simulink model "LabB_CheckCommunications"  (R2025b)
settings: Solver=FixedStepDiscrete  StartTime=0.0  StopTime=Inf  FixedStep=fSamplingPeriod  RelTol=1e-3  EnableMultiTasking=on
values from neighbouring files (symbols this model uses):
  fSamplingPeriod = 0.01    [GetDataFromSerial.m]    (also in GetRuns.m = 0.005; LabA_Solutions_LoadPhysicalParameters.m = 1 / sampling_freq; LabA_solutions.m = 1 / sampling_freq; LabB_ObserverAndControllerOverRobot_Parameters.m = 0.005)
undefined symbols (not defined in the file or in its folder): DiscIntNeverNeededParam
libraries: simulink_extras x3, arduinolib x3, xpcutilitieslib x1, MinSegLibrary_M2V3 x1
settings Model: SimulationMode=external  ExtModeTrigDuration=2  Creator=Alec  LastModifiedBy=emil
settings SolverCC: AlgebraicLoopSolver=TrustRegion
settings DataIOCC: LimitDataPoints=on  SaveFormat=Array  ReturnWorkspaceOutputs=off
settings OptimizationCC: PassReuseOutputArgsAs=Individual arguments  ExpressionDepthLimit=2147483647.0  MaxStackSize=64  EfficientTunableParamExpr=on
settings DebuggingCC: UnderspecifiedInitializationDetection=Classic  MergeDetectMultiDrivingBlocksExec=none  ParameterTunabilityLossMsg=error  UnconnectedInputMsg=warning  UnconnectedOutputMsg=warning  UnconnectedLineMsg=warning  StateNameClashWarn=warning  SFUnexpectedBacktrackingDiag=warning  SFNoUnconditionalDefaultTransitionDiag=warning  SFExecutionAtInitializationDiag=none  ArithmeticOperatorsInVariantConditions=warning
settings HardwareCC: ProdBitPerInt=16.0  ProdBitPerPointer=16.0  ProdBitPerSizeT=16.0  ProdBitPerPtrDiffT=16.0  ProdLargestAtomicFloat=None  ProdWordSize=8.0  ProdHWDeviceType=Atmel->AVR
settings ModelReferenceCC: EnableRefExpFcnMdlSchedulingChecks=on  PropagateSignalLabelsOutOfModel=off
settings SFSimCC: SimUseLocalCustomCode=off  MATLABDynamicMemAlloc=off  CustomCodeUndefinedFunction=UseInterfaceOnly
settings RTWCC: SystemTargetFile=ert.tlc  HardwareBoard=Arduino Mega 2560  TemplateMakefile=ert_default_tmf  GenerateReport=on  RTWVerbose=off  RTWUseLocalCustomCode=off  Toolchain=Arduino AVR  BuildConfiguration=Faster Runs  IncludeHyperlinkInReport=on  LaunchReport=on  GenerateTraceInfo=on  GenerateTraceReport=on  GenerateTraceReportSl=on  GenerateTraceReportSf=on  GenerateTraceReportEml=on  GPUComputeCapability=3.5  Description=Embedded Coder
settings CodeAppCC: ForceParamTrailComments=on  IgnoreCustomStorageClasses=off  OperatorAnnotations=on  SimulinkDataObjDesc=on  SFDataObjDesc=on  MATLABFcnDesc=on  CustomSymbolStrType=$N$R$M  InsertBlockDesc=on  StateflowObjectComments=on  MATLABSourceComments=on  InternalIdentifier=Classic
settings ERTTargetCC: InlinedParameterPlacement=Hierarchical  DynamicArrayContainerType=coder::array  SupportContinuousTime=on  SupportVariableSizeSignals=on
settings ConfigComp: CovMetricSettings=dw  CovSaveCumulativeToWorkspaceVar=on  CovSaveSingleToWorkspaceVar=on  CovExternalEMLEnable=off

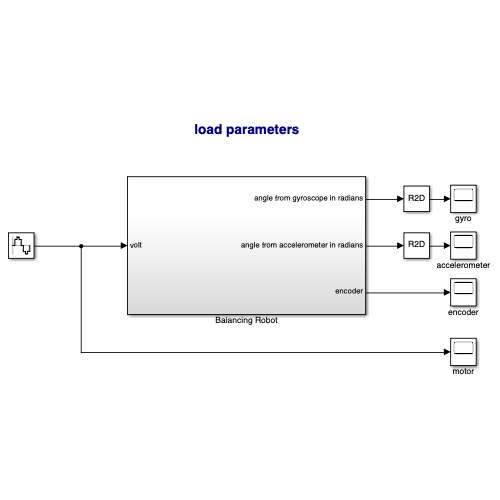
[thumbnail: Simulink's stored preview of the top-level diagram]
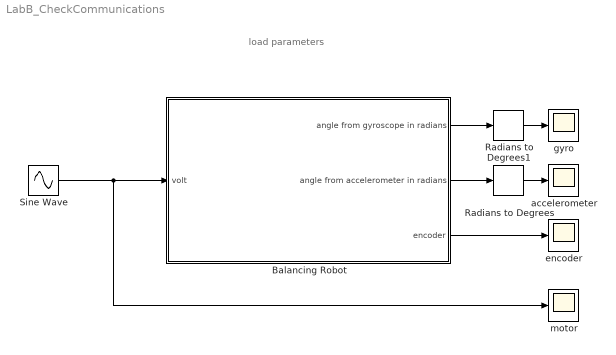
== system LabB_CheckCommunications ==
  note: load parameters
  Balancing Robot : Subsystem
  Radians to Degrees : simulink_extras/Transformations/Radians to Degrees
  Radians to Degrees1 : simulink_extras/Transformations/Radians to Degrees
  Sine Wave : Sin  Frequency=5  SampleTime=fSamplingPeriod
  accelerometer : Scope
      settings: ActiveDisplayYMinimum=-45  ActiveDisplayYMaximum=30  DataLoggingVariableName=tAngleFromAccelerometer
  encoder : Scope
      settings: TimeSpan=10  ActiveDisplayYMinimum=-268.25  ActiveDisplayYMaximum=-125.75  DataLoggingVariableName=tEncoder
  gyro : Scope
      settings: ActiveDisplayYMinimum=16.70976  ActiveDisplayYMaximum=26.00492  DataLoggingVariableName=tAngleFromGyro
  motor : Scope
      settings: ActiveDisplayYMinimum=-1  ActiveDisplayYMaximum=1  DataLoggingVariableName=tMotor
  wires:
  Balancing Robot/1(angle from gyroscope in radians) -> Radians to Degrees1/1
  Balancing Robot/2(angle from accelerometer in radians) -> Radians to Degrees/1
  Balancing Robot/3(encoder) -> encoder/1
  Radians to Degrees1/1 -> gyro/1
  Radians to Degrees/1 -> accelerometer/1
  Sine Wave/1 -> motor/1, Balancing Robot/1(volt)

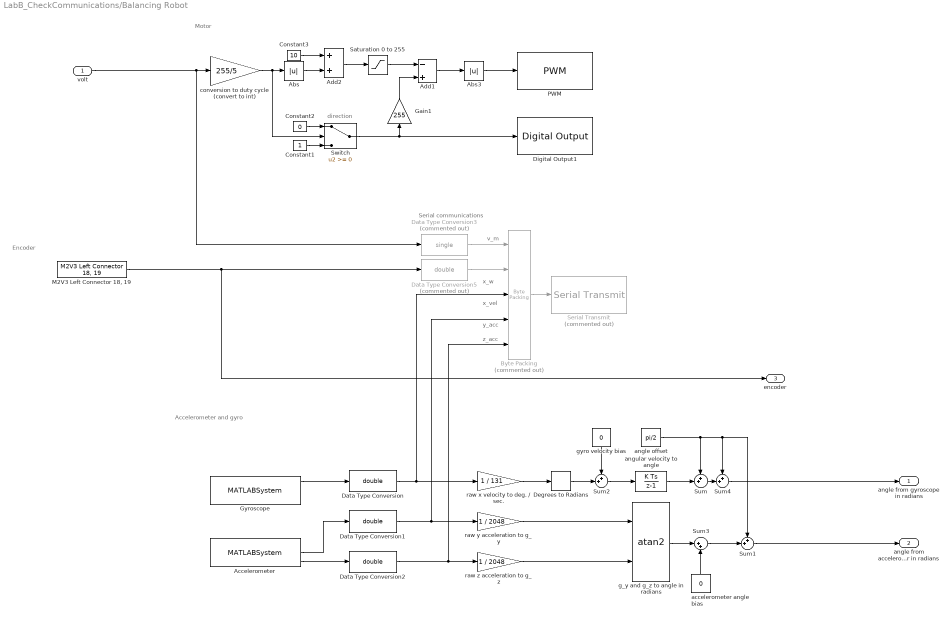
== system LabB_CheckCommunications/Balancing Robot ==
  note: v_m
  note: direction
  note: Encoder
  note: Accelerometer and gyro
  note: Motor
  note: Serial communications
  note: x_w
  note: x_vel
  note: y_acc
  note: z_acc
  volt : Inport
  Abs : Abs  SaturateOnIntegerOverflow=off
  Abs3 : Abs  SaturateOnIntegerOverflow=off
  Accelerometer : MATLABSystem  System=soMPU6050Accel  SimulateUsing=Code generation
      mask Type: soMPU6050Accel
  Add1 : Sum  Inputs=-+
  Add2 : Sum
  "Byte Packing " : xpcutilitieslib/Byte Packing   Commented=on  MaskPackedDataType=uint8  MaskUnpackedDataTypes={'single','double','double','double','double'}  MaskAlignment=1
  Constant1 : Constant
  Constant2 : Constant  Value=0
  Constant3 : Constant  Value=10
  Data Type Conversion : DataTypeConversion  OutDataTypeStr=double  SaturateOnIntegerOverflow=off  RndMeth=Floor
  Data Type Conversion1 : DataTypeConversion  OutDataTypeStr=double  SaturateOnIntegerOverflow=off  RndMeth=Floor
  Data Type Conversion2 : DataTypeConversion  OutDataTypeStr=double  SaturateOnIntegerOverflow=off  RndMeth=Floor
  Data Type Conversion3 : DataTypeConversion  Commented=on  OutDataTypeStr=single  SaturateOnIntegerOverflow=off  RndMeth=Floor
  Data Type Conversion5 : DataTypeConversion  Commented=on  OutDataTypeStr=double  SaturateOnIntegerOverflow=off  RndMeth=Floor
  Degrees to Radians : simulink_extras/Transformations/Degrees to Radians
  Digital Output1 : arduinolib/Digital Output  pinNumber=6  Direction=output  blockPlatform=arduino
  Gain1 : Gain  Gain=255
  Gyroscope : MATLABSystem  System=soMPU6050Gyro  DLPFmode=0
      mask Type: soMPU6050Gyro
  "M2V3 Left Connector 18, 19" : MinSegLibrary_M2V3/M2V3 Left Connector 18, 19  Encoder=1  PinA=19  PinB=18
      settings: SourceProductName=M2V3.2 Library
  PWM : arduinolib/PWM  pinNumber=8  frequencyType=Default  desiredFrequency=490.2  achievableFrequency=490.2
  Saturation 0 to 255 : Saturate  UpperLimit=255  LowerLimit=0
  Serial Transmit : arduinolib/Serial Transmit  Commented=on  portNumber=0  sendmode=write  sendformat=Decimal  floatprecision=2  blockPlatform=arduino
      settings: SourceProductName=Simulink Support Package for Arduino Hardware
  Sum{,1..2,4} (4 alike) : Sum  Inputs=++|
  Sum3 : Sum  Inputs=|++
  Switch : Switch  SaturateOnIntegerOverflow=off  InputSameDT=off
  accelerometer angle bias : Constant  Value=0
  angle offset : Constant  Value=pi/2
  angular velocity to angle : DiscreteIntegrator  SampleTime=-1  ICPrevOutput=DiscIntNeverNeededParam  ICPrevScaledInput=DiscIntNeverNeededParam
  conversion to duty cycle (convert to int) : Gain  Gain=255/5  OutDataTypeStr=int16
  g_y and g_z to angle in radians : Trigonometry  Operator=atan2
  gyro velocity bias : Constant  Value=0
  raw x velocity to deg. / sec. : Gain  Gain=1 / 131
  raw y acceleration to g_y : Gain  Gain=1 / 2048
  raw z acceleration to g_z : Gain  Gain=1 / 2048
  angle from gyroscope in radians : Outport
  angle from accelerometer in radians : Outport  Port=2
  encoder : Outport  Port=3
  wires:
  Gyroscope/1 -> Data Type Conversion/1
  Accelerometer/2 -> Data Type Conversion1/1
  raw z acceleration to g_z/1 -> g_y and g_z to angle in radians/2
  raw y acceleration to g_y/1 -> g_y and g_z to angle in radians/1
  angle offset/1 -> Sum4/1, Sum1/1, Sum/1
  raw x velocity to deg. / sec./1 -> Degrees to Radians/1
  Sum/1 -> Sum4/2
  Data Type Conversion2/1 -> "Byte Packing "/5, raw z acceleration to g_z/1
  Data Type Conversion1/1 -> "Byte Packing "/4, raw y acceleration to g_y/1
  Data Type Conversion/1 -> "Byte Packing "/3, raw x velocity to deg. / sec./1
  Accelerometer/3 -> Data Type Conversion2/1
  Add2/1 -> Saturation 0 to 255/1
  Abs/1 -> Add2/2
  Constant3/1 -> Add2/1
  Abs3/1 -> PWM/1
  Saturation 0 to 255/1 -> Add1/1
  conversion to duty cycle (convert to int)/1 -> Abs/1, Switch/2
  Add1/1 -> Abs3/1
  Gain1/1 -> Add1/2
  Constant1/1 -> Switch/3
  Constant2/1 -> Switch/1
  Switch/1 -> Gain1/1, Digital Output1/1
  volt/1 -> Data Type Conversion3/1, conversion to duty cycle (convert to int)/1
  "Byte Packing "/1 -> Serial Transmit/1
  "M2V3 Left Connector 18, 19"/1 -> encoder/1, Data Type Conversion5/1
  Data Type Conversion3/1 -> "Byte Packing "/1
  Data Type Conversion5/1 -> "Byte Packing "/2
  Sum1/1 -> angle from accelerometer in radians/1
  angular velocity to angle/1 -> Sum/2
  Degrees to Radians/1 -> Sum2/2
  gyro velocity bias/1 -> Sum2/1
  Sum2/1 -> angular velocity to angle/1
  g_y and g_z to angle in radians/1 -> Sum3/1
  Sum3/1 -> Sum1/2
  accelerometer angle bias/1 -> Sum3/2
  Sum4/1 -> angle from gyroscope in radians/1
